simulink model "sm_robotic_wrist"  (R2021b)
settings: Solver=ode15s  StartTime=0.0  StopTime=10  FixedStep=1e-3  MaxStep=0.1  RelTol=1e-4  AbsTol=1e-4  EnableMultiTasking=on
model workspace: external: MATLAB File sm_robotic_wrist_params.m (data not in the file)
values from neighbouring files (symbols this model uses):
  Ca = 60    [sm_robotic_wrist_params.m]
  color = simmechanics.demohelpers.colors    [sm_robotic_wrist_params.m]
  density = simmechanics.demohelpers.densities    [sm_robotic_wrist_params.m]
undefined symbols (not defined in the file or in its folder): forearm, prcarrier, prshaft, tassm, trcarrier, trshaft, wshaft, X, Y, Z
libraries: sm_lib x44, sm_robotic_wrist_lib x12, nesl_utility x4
(part 1 of 2)
Description:
  | 3-Roll Robotic Wrist Mechanism
  | 
  | This example models a 3-Roll robotic wrist mechanism based on the Cincinnati-Milacron 3-roll wrist mechanism. The mechanism uses three bevel gear pairs to rotate the tool about 3 independent axes. The tip of the tool moves along the surface of a sphere and can be rotated about an axis that passes through the center of that sphere (drilling action). In this example, precomputed torques are applied to the three drive shafts to achieve a certain trajectory (on the surface of the sphere) of the tool tip. Drilling is performed at different points along the trajectory.
settings Model: Creator=The MathWorks, Inc.  LastModifiedBy=The MathWorks, Inc.
settings SolverCC: AutoScaleAbsTol=off  AlgebraicLoopSolver=TrustRegion
settings DataIOCC: LimitDataPoints=on  SaveFormat=Array  SaveOutput=off  SaveTime=off  ReturnWorkspaceOutputs=off
settings OptimizationCC: LifeSpan=inf
settings DebuggingCC: UnderspecifiedInitializationDetection=Classic  MergeDetectMultiDrivingBlocksExec=none  SFUnexpectedBacktrackingDiag=warning  SFNoUnconditionalDefaultTransitionDiag=warning  SFExecutionAtInitializationDiag=none  SFMachineParentedDataDiag=warning  ArithmeticOperatorsInVariantConditions=warning
settings HardwareCC: ProdBitPerPointer=32  ProdBitPerSizeT=32  ProdBitPerPtrDiffT=32  ProdLargestAtomicFloat=None  ProdIntDivRoundTo=Undefined  ProdEndianess=Unspecified  ProdWordSize=32  ProdHWDeviceType=32-bit Generic
settings ModelReferenceCC: PropagateSignalLabelsOutOfModel=off
settings SFSimCC: SimUseLocalCustomCode=off  CustomCodeUndefinedFunction=UseInterfaceOnly
settings RTWCC: RTWUseLocalCustomCode=off
settings CodeAppCC: StateflowObjectComments=on
settings GRTTargetCC: TargetLangStandard=C89/C90 (ANSI)
settings ConfigComp: CovMetricSettings=dw  CovSaveCumulativeToWorkspaceVar=on  CovSaveSingleToWorkspaceVar=on  CovExternalEMLEnable=off
settings SimscapeCC: SimscapeNormalizeSystem=off
settings ConfigurationSet: Description=SimMechanics 2G
settings ExplorerConfigSet: InternalSimMechanicsExplorerSettings="<ExplorerConfiguration><canonicalview>default</canonicalview><TilePanel><TileInfo><Tiles Columns=\"1\" Count=\"1\" Rows=\"1\"><Column Left=\"2\" Weight=\"1\"/><Column Left=\"812\"/><Row Top=\"2\" Weight=\"1\"/><Row Top=\"689\"/><Tile Height=\"1\" Width=\"1\" X=\"0\" Y=\"0\"/></Tiles></TileInfo><SceneInfo><SceneViewer><BGColor><R>0.60000002384185791</R><G>0.60000002384185791</G><B>0.60000002384185791</B></BGColor><Camera><Position><X>0.167588576674461365</X><Y>-0.43597028678660954</Y><Z>1.21854245662689209e-05</Z></Position><Center><X>0.167588576674461365</X><Y>1.28261744976043701e-05</Y><Z>1.21854245662689209e-05</Z></Center><Up><X>0</X><Y>-0</Y><Z>1</Z></Up><Left>-0.17596800550818445</Left><Right>0.17596800550818445</Right><Bottom>-0.0837415538728237124</Bottom><Top>0.0837415538728237124</Top></Camera></SceneViewer></SceneInfo></TilePanel></ExplorerConfiguration>"

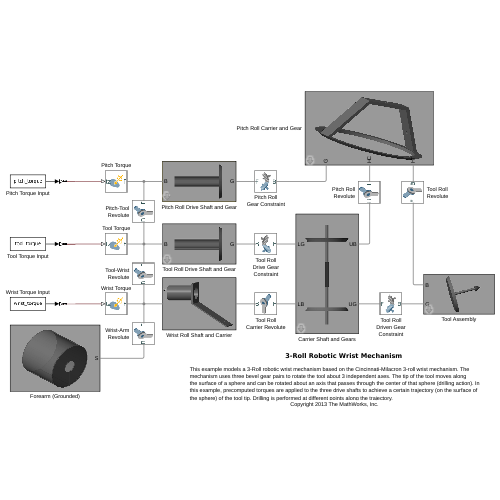
[thumbnail: Simulink's stored preview of the top-level diagram]
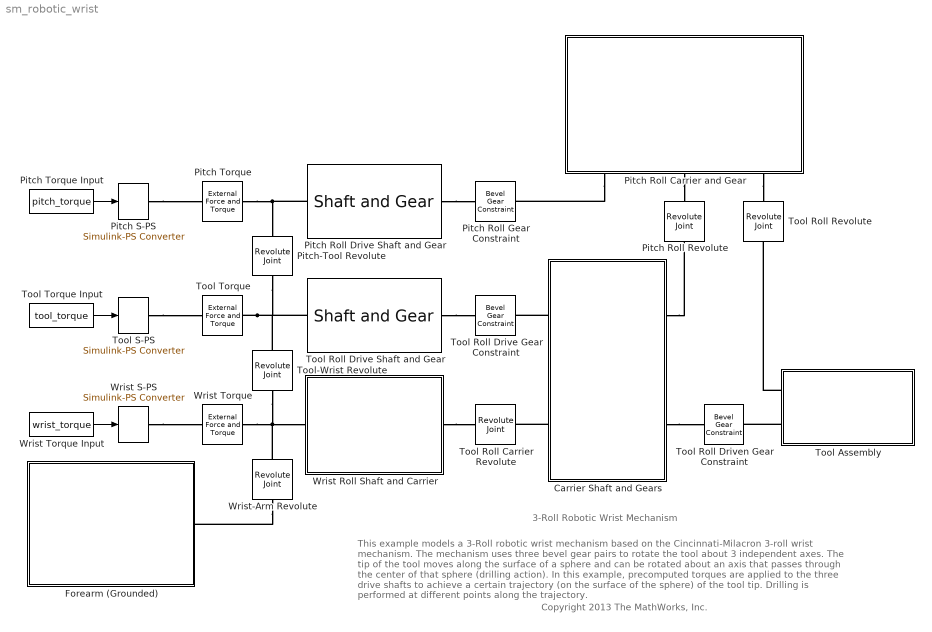
== system sm_robotic_wrist ==
  note: 3-Roll Robotic Wrist Mechanism
  note: Copyright 2013 The MathWorks, Inc.
  note: This example models a 3-Roll robotic wrist mechanism based on the Cincinnati-Milacron 3-roll wrist mechanism. The
      | mechanism uses three bevel gear pairs to rotate the tool about 3 independent axes. The tip of the tool moves along
      | the surface of a sphere and can be rotated about an axis that passes through the center of that sphere (drilling action). In
      | this example, precomputed torques are applied to the three drive shafts to achieve a certain trajectory (on the surface of
      | the sphere) of the tool tip. Drilling is performed at different points along the trajectory.
  Carrier Shaft and Gears : Subsystem  mask(Tool Roll Carrier){R=trcarrier.Rs, L=trcarrier.Ls, Og=trcarrier.Og, Ohl=trcarrier.Olb, Ohu=trcarrier.Oub, Rg=trcarrier.Rg, Tg=trcarrier.Tg, Ca=90-Ca, Hg=trcarrier.Rgh, rho=density.aluminum, clr=color.yellow}
      mask prompts: R "Radius (cm):"; L "Length (cm):"; Og "Gear offset (cm):"; Ohl "Lower hinge offset (cm):"; Ohu "Upper hinge offset (cm):"; Rg "Gear radius (cm):"; Tg "Gear thickness (cm):"; Ca "Gear cone angle (deg):"; Hg "Gear hole radius (cm):"; rho "Density (kg/m^3)"; clr "Color [r g b]:"
      mask help:
      | This block models the intermediate carrier (with bevel gears) that transmits the torque from the tool roll drive shaft to the tool.
      |
      | The port LG and UG correspond to the frames of the lower and upper gears.
      |
      | The port LB and UB correspond to the frames of the lower and upper bearing points.
      mask DialogControl Container4 Prompt: Shaft
      mask DialogControl Container4_copy_copy Prompt: Gears
      mask DialogControl Container4_copy Prompt: Material Properties
      mask Display:
      | image(fullfile(matlabroot,'toolbox','physmod','sm','smdemos','robotic_wrist','images','sm_rwrist_toolrollcarrier.png'))
      | port_label('LConn',1,'LG')
      | port_label('LConn',2,'LB')
      | port_label('RConn',1,'UB')
      | port_label('RConn',2,'UG')
  Forearm (Grounded) : Subsystem
      mask Display:
      | image(fullfile(matlabroot,'toolbox','physmod','sm','smdemos','robotic_wrist','images','sm_rwrist_forearm.png'))
      | port_label('RConn',1,'S')
  Pitch Roll Gear Constraint : sm_lib/Gears and Couplings/Gears/Bevel Gear Constraint  BaseGearRadius=prcarrier.Rg  BaseGearRadiusUnits=cm  FollGearRadius=prshaft.Rg  FollGearRadiusUnits=cm  AssemblyGearRotation=Free  ShaftOrientation=ArbitrarilyOriented  ShaftAngle=180-Ca  ShaftAngleUnits=deg
      settings: SourceProductBaseCode=MS
  Pitch Roll Revolute : sm_lib/Joints/Revolute Joint  JointMode=Normal  SenseConstraintForce=off  SenseConstraintForceX=off  SenseConstraintForceY=off  SenseConstraintForceZ=off  SenseConstraintTorque=off  SenseConstraintTorqueX=off  SenseConstraintTorqueY=off  SenseConstraintTorqueZ=off  SenseTotalForce=off  SenseTotalForceX=off  SenseTotalForceY=off  SenseTotalForceZ=off  SenseTotalTorque=off  SenseTotalTorqueX=off  SenseTotalTorqueY=off  SenseTotalTorqueZ=off  CompositeWrenchDir=FollowerOnBase  CompositeWrenchFrame=BaseFrame  EquilibriumPosition=0  EquilibriumPositionUnits=deg  SpringStiffness=0  SpringStiffnessUnits=N*m/deg  DampingCoefficient=0  DampingCoefficientUnits=N*m/(deg/s)  TorqueActuationMode=NoTorque  MotionActuationMode=ComputedMotion  SensePosition=off  SenseVelocity=off  SenseAcceleration=off  SenseTorqueForce=off  SenseLowerLimitTorqueForce=off  SenseUpperLimitTorqueForce=off  LowerLimitSpecify=off  LowerLimitBound=-90  LowerLimitBoundUnits=deg  LowerLimitStiffness=1e4  LowerLimitStiffnessUnits=N*m/deg  LowerLimitDamping=10  LowerLimitDampingUnits=N*m/(deg/s)  LowerLimitTransitionRegionWidth=0.1  LowerLimitTransitionRegionWidthUnits=deg  UpperLimitSpecify=off  UpperLimitBound=90  UpperLimitBoundUnits=deg  UpperLimitStiffness=1e4  UpperLimitStiffnessUnits=N*m/deg  UpperLimitDamping=10  UpperLimitDampingUnits=N*m/(deg/s)  UpperLimitTransitionRegionWidth=0.1  UpperLimitTransitionRegionWidthUnits=deg  PositionTargetSpecify=on  PositionTargetPriority=High  PositionTargetValue=joint_targets.pitch_roll.q  PositionTargetValueUnits=rad  VelocityTargetSpecify=on  VelocityTargetPriority=High  VelocityTargetValue=joint_targets.pitch_roll.w  VelocityTargetValueUnits=rad/s
  Pitch Roll Carrier and Gear : Subsystem  mask(Pitch Roll Carrier){Hc=prcarrier.Hc, Ac=Ca, Tc=prcarrier.Tc, Wc=prcarrier.Wc, Rht=prcarrier.Rht, Rhc=prcarrier.Rhc, Rg=prcarrier.Rg, Tg=prcarrier.Tg, Rgh=prcarrier.Rgh, Ag=Ca, rho=density.aluminum, cclr=color.brown, gclr=color.brown}
      mask prompts: Hc "Carrier height (cm):"; Ac "Carrier arms angle (deg):"; Tc "Carrier arms thickness (cm):"; Wc "Carrier arms width (cm):"; Rht "Tool shaft hole radius (cm):"; Rhc "Carrier shaft hole radius (cm):"; Rg "Gear radius (cm):"; Tg "Gear thickness (cm):"; Rgh "Gear hole radius (cm):"; Ag "Gear cone angle (deg):"; rho "Density (kg/m^3):"; cclr "Carrier color [r g b]:"; gclr "Gear color [r g b]:"
      mask help:
      | This block models the pitch roll carrier and gear that carries the tool and rotates the tool about the pitch axis. The bevel gear is welded to the carrier and is driven by the pitch roll drive shaft.
      |
      | The port G corresponds to the center of the bevel gear.
      |
      | The port HC corresponds to the bearing between the pitch carrier and the tool roll carrier.
      |
      | The port HT correponds to the bearing between the pitch carrier and the tool assembly.
      mask init:
      | sn = sin(Ac*pi/180);
      | tn = tan(Ac*pi/180);
      | 
      | sn1 = sin((90-Ac)*pi/180);
      | cn1 = cos((90-Ac)*pi/180);
      | 
      | w = Tc/sn;
      | Oht = (Hc-Tc)/sn - (Rg-w/2)*sn1 + Tg*sn/2;
      | 
      | carrier_left_xsec = [-2*Rhc             Hc
      |                     -Rg-w/2+Hc/tn      Hc;
      |                     -Rg-w/2            0;
      |                     -Rg+w/2            0;
      |                     -Rg+w/2+(Hc-Tc)/tn Hc-Tc;
      |                     -2*Rhc             Hc-Tc];
      |                 
      | carrier_right_top_xsec = ...
      |      [2*Rhc                                     Hc-Tc;
      |       Rg-w/2-(Hc-Tc)/tn                         Hc-Tc;
      |       Rg-w/2-(Hc-Tc)/tn+(Oht-2*Rht)*sn1         Hc-Tc-(Oht-2*Rht)*cn1;
      |       Rg-w/2-(Hc-Tc)/tn+(Oht-2*Rht)*sn1+Tc*cn1  Hc-Tc-(Oht-2*Rht)*cn1+Tc*sn1;
      |       Rg+w/2-Hc/tn                              Hc;
      |       2*Rhc                                     Hc
      |      ];
      |    
      | carrier_right_bot_xsec = ...
      |       [ Rg-w/2                                    0;
      |         Rg+w/2                                    0;
      |         Rg-w/2-(Hc-Tc)/tn+(Oht+2*Rht)*sn1+Tc*cn1  Hc-Tc-(Oht+2*Rht)*cn1+Tc*sn1;
      |         Rg-w/2-(Hc-Tc)/tn+(Oht+2*Rht)*sn1         Hc-Tc-(Oht+2*Rht)*cn1
      |       ];
      |   
      | rhx = Rg-w/2-(Hc-Tc)/tn+Oht*sn1;
      | rhy = Hc-Tc -Oht*cn1;
      mask DialogControl Container4 Prompt: Carrier Arm
      mask DialogControl Container4_copy Prompt: Gear
      mask DialogControl Container4_copy_copy Prompt: Material Properties
      mask Display:
      | image(fullfile(matlabroot,'toolbox','physmod','sm','smdemos','robotic_wrist','images','sm_rwrist_pitchrollcarrier.png'))
      | port_label('RConn',1,'G')
      | port_label('RConn',2,'HC')
      | port_label('RConn',3,'HT')
  Pitch Roll Drive Shaft and Gear : sm_robotic_wrist_lib/Shaft and Gear  L=prshaft.Ls  Ro=prshaft.Rso  Ri=prshaft.Rsi  Rg=prshaft.Rg  Tg=prshaft.Tg  Cag=Ca  rho=density.aluminum  clr=color.brown  Os=1
      settings: SourceProductBaseCode=MS
  Pitch S-PS : nesl_utility/Simulink-PS Converter  PhysicalDomain=network_engine_domain  SubClassName=ps_input  LeftPortType=input  RightPortType=output  PseudoPeriodic=off  Frequencies=[]  NoiseDistribution=none  NoiseParameters=[]  Unit=1  AffineConversion=off  FilteringAndDerivatives=filter  SimscapeFilterOrder=2  InputFilterTimeConstant=0.01  UdotUserProvided=1
      settings: SourceProductBaseCode=PW,SS
  Pitch Torque : sm_lib/Forces and Torques/External Force and Torque  ForceResolutionFrame=AttachedFrame  EnableForceX=off  EnableForceY=off  EnableForceZ=off  EnableForce=off  TorqueResolutionFrame=AttachedFrame  EnableTorqueX=off  EnableTorqueY=off  EnableTorqueZ=on  EnableTorque=off
  Pitch Torque Input : FromWorkspace  VariableName=pitch_torque
  Pitch-Tool Revolute : sm_lib/Joints/Revolute Joint  JointMode=Normal  SenseConstraintForce=off  SenseConstraintForceX=off  SenseConstraintForceY=off  SenseConstraintForceZ=off  SenseConstraintTorque=off  SenseConstraintTorqueX=off  SenseConstraintTorqueY=off  SenseConstraintTorqueZ=off  SenseTotalForce=off  SenseTotalForceX=off  SenseTotalForceY=off  SenseTotalForceZ=off  SenseTotalTorque=off  SenseTotalTorqueX=off  SenseTotalTorqueY=off  SenseTotalTorqueZ=off  CompositeWrenchDir=FollowerOnBase  CompositeWrenchFrame=BaseFrame  EquilibriumPosition=0  EquilibriumPositionUnits=deg  SpringStiffness=0  SpringStiffnessUnits=N*m/deg  DampingCoefficient=5e-3  DampingCoefficientUnits=N*m/(deg/s)  TorqueActuationMode=NoTorque  MotionActuationMode=ComputedMotion  SensePosition=off  SenseVelocity=off  SenseAcceleration=off  SenseTorqueForce=off  SenseLowerLimitTorqueForce=off  SenseUpperLimitTorqueForce=off  LowerLimitSpecify=off  LowerLimitBound=-90  LowerLimitBoundUnits=deg  LowerLimitStiffness=1e4  LowerLimitStiffnessUnits=N*m/deg  LowerLimitDamping=10  LowerLimitDampingUnits=N*m/(deg/s)  LowerLimitTransitionRegionWidth=0.1  LowerLimitTransitionRegionWidthUnits=deg  UpperLimitSpecify=off  UpperLimitBound=90  UpperLimitBoundUnits=deg  UpperLimitStiffness=1e4  UpperLimitStiffnessUnits=N*m/deg  UpperLimitDamping=10  UpperLimitDampingUnits=N*m/(deg/s)  UpperLimitTransitionRegionWidth=0.1  UpperLimitTransitionRegionWidthUnits=deg  PositionTargetSpecify=on  PositionTargetPriority=High  PositionTargetValue=joint_targets.pitch_tool.q  PositionTargetValueUnits=rad  VelocityTargetSpecify=on  VelocityTargetPriority=High  VelocityTargetValue=joint_targets.pitch_tool.w  VelocityTargetValueUnits=rad/s
  Tool Assembly : Subsystem  mask(Tool Assembly){L=tassm.Ls, R=tassm.Rs, Oh=tassm.Ohs, Rd=tassm.Rd, Hd=tassm.Hd, Rg=tassm.Rg, Tg=tassm.Tg, Cag=90-Ca, rho=density.aluminum, clr=color.yellow}
      mask prompts: L "Shaft length (cm):"; R "Shaft radius (cm):"; Oh "Hinge offset (cm):"; Rd "Drill base radius (cm):"; Hd "Drill height (cm):"; Rg "Gear radius (cm):"; Tg "Gear thickness (cm):"; Cag "Gear cone angle (deg):"; rho "Density (kg/m^3):"; clr "Color [r g b]:"
      mask help:
      | This block models the drill tool and the attached bevel gear. The bevel gear is driven by the tool roll gear train.
      |
      | The port G corresponds to the frame at the center of the bevel gear.
      |
      | The port B corresponds to the frame at the pitch roll carrier bearing.
      mask init:
      | drill_xsec = [0 0; Rd 0; 0 Hd];
      mask DialogControl Container4 Prompt: Tool
      mask DialogControl Container4_copy Prompt: Gear
      mask DialogControl Container4_copy_copy Prompt: Material Properties
      mask Display:
      | image(fullfile(matlabroot,'toolbox','physmod','sm','smdemos','robotic_wrist','images','sm_rwrist_toolassm.png'))
      | port_label('LConn',1,'B')
      | port_label('LConn',2,'G')
  Tool Roll Carrier Revolute : sm_lib/Joints/Revolute Joint  JointMode=Normal  SenseConstraintForce=off  SenseConstraintForceX=off  SenseConstraintForceY=off  SenseConstraintForceZ=off  SenseConstraintTorque=off  SenseConstraintTorqueX=off  SenseConstraintTorqueY=off  SenseConstraintTorqueZ=off  SenseTotalForce=off  SenseTotalForceX=off  SenseTotalForceY=off  SenseTotalForceZ=off  SenseTotalTorque=off  SenseTotalTorqueX=off  SenseTotalTorqueY=off  SenseTotalTorqueZ=off  CompositeWrenchDir=FollowerOnBase  CompositeWrenchFrame=BaseFrame  EquilibriumPosition=0  EquilibriumPositionUnits=deg  SpringStiffness=0  SpringStiffnessUnits=N*m/deg  DampingCoefficient=0  DampingCoefficientUnits=N*m/(deg/s)  TorqueActuationMode=NoTorque  MotionActuationMode=ComputedMotion  SensePosition=off  SenseVelocity=off  SenseAcceleration=off  SenseTorqueForce=off  SenseLowerLimitTorqueForce=off  SenseUpperLimitTorqueForce=off  LowerLimitSpecify=off  LowerLimitBound=-90  LowerLimitBoundUnits=deg  LowerLimitStiffness=1e4  LowerLimitStiffnessUnits=N*m/deg  LowerLimitDamping=10  LowerLimitDampingUnits=N*m/(deg/s)  LowerLimitTransitionRegionWidth=0.1  LowerLimitTransitionRegionWidthUnits=deg  UpperLimitSpecify=off  UpperLimitBound=90  UpperLimitBoundUnits=deg  UpperLimitStiffness=1e4  UpperLimitStiffnessUnits=N*m/deg  UpperLimitDamping=10  UpperLimitDampingUnits=N*m/(deg/s)  UpperLimitTransitionRegionWidth=0.1  UpperLimitTransitionRegionWidthUnits=deg  PositionTargetSpecify=off  PositionTargetPriority=High  PositionTargetValue=-2.786559909696359e+00  PositionTargetValueUnits=deg  VelocityTargetSpecify=off  VelocityTargetPriority=High  VelocityTargetValue=0  VelocityTargetValueUnits=deg/s
  Tool Roll Drive Gear Constraint : sm_lib/Gears and Couplings/Gears/Bevel Gear Constraint  BaseGearRadius=trshaft.Rg  BaseGearRadiusUnits=cm  FollGearRadius=trcarrier.Rg  FollGearRadiusUnits=cm  AssemblyGearRotation=Free  ShaftOrientation=ArbitrarilyOriented  ShaftAngle=Ca  ShaftAngleUnits=deg
      settings: SourceProductBaseCode=MS
  Tool Roll Driven Gear Constraint : sm_lib/Gears and Couplings/Gears/Bevel Gear Constraint  BaseGearRadius=tassm.Rg  BaseGearRadiusUnits=cm  FollGearRadius=trcarrier.Rg  FollGearRadiusUnits=cm  AssemblyGearRotation=Free  ShaftOrientation=ArbitrarilyOriented  ShaftAngle=Ca  ShaftAngleUnits=deg
      settings: SourceProductBaseCode=MS
  Tool Roll Revolute : sm_lib/Joints/Revolute Joint  JointMode=Normal  SenseConstraintForce=off  SenseConstraintForceX=off  SenseConstraintForceY=off  SenseConstraintForceZ=off  SenseConstraintTorque=off  SenseConstraintTorqueX=off  SenseConstraintTorqueY=off  SenseConstraintTorqueZ=off  SenseTotalForce=off  SenseTotalForceX=off  SenseTotalForceY=off  SenseTotalForceZ=off  SenseTotalTorque=off  SenseTotalTorqueX=off  SenseTotalTorqueY=off  SenseTotalTorqueZ=off  CompositeWrenchDir=FollowerOnBase  CompositeWrenchFrame=BaseFrame  EquilibriumPosition=0  EquilibriumPositionUnits=deg  SpringStiffness=0  SpringStiffnessUnits=N*m/deg  DampingCoefficient=0  DampingCoefficientUnits=N*m/(deg/s)  TorqueActuationMode=NoTorque  MotionActuationMode=ComputedMotion  SensePosition=off  SenseVelocity=off  SenseAcceleration=off  SenseTorqueForce=off  SenseLowerLimitTorqueForce=off  SenseUpperLimitTorqueForce=off  LowerLimitSpecify=off  LowerLimitBound=-90  LowerLimitBoundUnits=deg  LowerLimitStiffness=1e4  LowerLimitStiffnessUnits=N*m/deg  LowerLimitDamping=10  LowerLimitDampingUnits=N*m/(deg/s)  LowerLimitTransitionRegionWidth=0.1  LowerLimitTransitionRegionWidthUnits=deg  UpperLimitSpecify=off  UpperLimitBound=90  UpperLimitBoundUnits=deg  UpperLimitStiffness=1e4  UpperLimitStiffnessUnits=N*m/deg  UpperLimitDamping=10  UpperLimitDampingUnits=N*m/(deg/s)  UpperLimitTransitionRegionWidth=0.1  UpperLimitTransitionRegionWidthUnits=deg  PositionTargetSpecify=off  PositionTargetPriority=High  PositionTargetValue=-4.321120546852593e+01  PositionTargetValueUnits=deg  VelocityTargetSpecify=off  VelocityTargetPriority=High  VelocityTargetValue=0  VelocityTargetValueUnits=deg/s
  Tool Roll Drive Shaft and Gear : sm_robotic_wrist_lib/Shaft and Gear  L=trshaft.Ls  Ro=trshaft.Rso  Ri=trshaft.Rsi  Rg=trshaft.Rg  Tg=trshaft.Tg  Cag=90-Ca  rho=density.aluminum  clr=color.yellow  Os=1
      settings: SourceProductBaseCode=MS
  Tool S-PS : nesl_utility/Simulink-PS Converter  PhysicalDomain=network_engine_domain  SubClassName=ps_input  LeftPortType=input  RightPortType=output  PseudoPeriodic=off  Frequencies=[]  NoiseDistribution=none  NoiseParameters=[]  Unit=1  AffineConversion=off  FilteringAndDerivatives=filter  SimscapeFilterOrder=2  InputFilterTimeConstant=0.01  UdotUserProvided=1
      settings: SourceProductBaseCode=PW,SS
  Tool Torque : sm_lib/Forces and Torques/External Force and Torque  ForceResolutionFrame=AttachedFrame  EnableForceX=off  EnableForceY=off  EnableForceZ=off  EnableForce=off  TorqueResolutionFrame=AttachedFrame  EnableTorqueX=off  EnableTorqueY=off  EnableTorqueZ=on  EnableTorque=off
  Tool Torque Input : FromWorkspace  VariableName=tool_torque
  Tool-Wrist Revolute : sm_lib/Joints/Revolute Joint  JointMode=Normal  SenseConstraintForce=off  SenseConstraintForceX=off  SenseConstraintForceY=off  SenseConstraintForceZ=off  SenseConstraintTorque=off  SenseConstraintTorqueX=off  SenseConstraintTorqueY=off  SenseConstraintTorqueZ=off  SenseTotalForce=off  SenseTotalForceX=off  SenseTotalForceY=off  SenseTotalForceZ=off  SenseTotalTorque=off  SenseTotalTorqueX=off  SenseTotalTorqueY=off  SenseTotalTorqueZ=off  CompositeWrenchDir=FollowerOnBase  CompositeWrenchFrame=BaseFrame  EquilibriumPosition=0  EquilibriumPositionUnits=deg  SpringStiffness=0  SpringStiffnessUnits=N*m/deg  DampingCoefficient=5e-3  DampingCoefficientUnits=N*m/(deg/s)  TorqueActuationMode=NoTorque  MotionActuationMode=ComputedMotion  SensePosition=off  SenseVelocity=off  SenseAcceleration=off  SenseTorqueForce=off  SenseLowerLimitTorqueForce=off  SenseUpperLimitTorqueForce=off  LowerLimitSpecify=off  LowerLimitBound=-90  LowerLimitBoundUnits=deg  LowerLimitStiffness=1e4  LowerLimitStiffnessUnits=N*m/deg  LowerLimitDamping=10  LowerLimitDampingUnits=N*m/(deg/s)  LowerLimitTransitionRegionWidth=0.1  LowerLimitTransitionRegionWidthUnits=deg  UpperLimitSpecify=off  UpperLimitBound=90  UpperLimitBoundUnits=deg  UpperLimitStiffness=1e4  UpperLimitStiffnessUnits=N*m/deg  UpperLimitDamping=10  UpperLimitDampingUnits=N*m/(deg/s)  UpperLimitTransitionRegionWidth=0.1  UpperLimitTransitionRegionWidthUnits=deg  PositionTargetSpecify=on  PositionTargetPriority=High  PositionTargetValue=joint_targets.tool_wrist.q  PositionTargetValueUnits=rad  VelocityTargetSpecify=on  VelocityTargetPriority=High  VelocityTargetValue=joint_targets.tool_wrist.w  VelocityTargetValueUnits=rad/s
  Wrist Roll Shaft and Carrier : Subsystem
      mask Display: image(fullfile(matlabroot,'toolbox','physmod','sm','smdemos','robotic_wrist','images','sm_rwrist_wristshaftcarrier.png'))
  Wrist S-PS : nesl_utility/Simulink-PS Converter  PhysicalDomain=network_engine_domain  SubClassName=ps_input  LeftPortType=input  RightPortType=output  PseudoPeriodic=off  Frequencies=[]  NoiseDistribution=none  NoiseParameters=[]  Unit=1  AffineConversion=off  FilteringAndDerivatives=filter  SimscapeFilterOrder=2  InputFilterTimeConstant=0.01  UdotUserProvided=1
      settings: SourceProductBaseCode=PW,SS
  Wrist Torque : sm_lib/Forces and Torques/External Force and Torque  ForceResolutionFrame=AttachedFrame  EnableForceX=off  EnableForceY=off  EnableForceZ=off  EnableForce=off  TorqueResolutionFrame=AttachedFrame  EnableTorqueX=off  EnableTorqueY=off  EnableTorqueZ=on  EnableTorque=off
  Wrist Torque Input : FromWorkspace  VariableName=wrist_torque
  Wrist-Arm Revolute : sm_lib/Joints/Revolute Joint  JointMode=Normal  SenseConstraintForce=off  SenseConstraintForceX=off  SenseConstraintForceY=off  SenseConstraintForceZ=off  SenseConstraintTorque=off  SenseConstraintTorqueX=off  SenseConstraintTorqueY=off  SenseConstraintTorqueZ=off  SenseTotalForce=off  SenseTotalForceX=off  SenseTotalForceY=off  SenseTotalForceZ=off  SenseTotalTorque=off  SenseTotalTorqueX=off  SenseTotalTorqueY=off  SenseTotalTorqueZ=off  CompositeWrenchDir=FollowerOnBase  CompositeWrenchFrame=BaseFrame  EquilibriumPosition=0  EquilibriumPositionUnits=deg  SpringStiffness=0  SpringStiffnessUnits=N*m/deg  DampingCoefficient=5e-3  DampingCoefficientUnits=N*m/(deg/s)  TorqueActuationMode=NoTorque  MotionActuationMode=ComputedMotion  SensePosition=off  SenseVelocity=off  SenseAcceleration=off  SenseTorqueForce=off  SenseLowerLimitTorqueForce=off  SenseUpperLimitTorqueForce=off  LowerLimitSpecify=off  LowerLimitBound=-90  LowerLimitBoundUnits=deg  LowerLimitStiffness=1e4  LowerLimitStiffnessUnits=N*m/deg  LowerLimitDamping=10  LowerLimitDampingUnits=N*m/(deg/s)  LowerLimitTransitionRegionWidth=0.1  LowerLimitTransitionRegionWidthUnits=deg  UpperLimitSpecify=off  UpperLimitBound=90  UpperLimitBoundUnits=deg  UpperLimitStiffness=1e4  UpperLimitStiffnessUnits=N*m/deg  UpperLimitDamping=10  UpperLimitDampingUnits=N*m/(deg/s)  UpperLimitTransitionRegionWidth=0.1  UpperLimitTransitionRegionWidthUnits=deg  PositionTargetSpecify=on  PositionTargetPriority=High  PositionTargetValue=joint_targets.wrist_arm.q  PositionTargetValueUnits=rad  VelocityTargetSpecify=on  VelocityTargetPriority=High  VelocityTargetValue=joint_targets.wrist_arm.w  VelocityTargetValueUnits=rad/s
  wires:
  Pitch Torque Input/1 -> Pitch S-PS/1
  Wrist Torque Input/1 -> Wrist S-PS/1
  Tool Torque Input/1 -> Tool S-PS/1
  connections:
  Wrist Torque/RConn1 -- Wrist-Arm Revolute/RConn1 -- Wrist Roll Shaft and Carrier/LConn1 -- Tool-Wrist Revolute/LConn1
  Pitch Torque/RConn1 -- Pitch Roll Drive Shaft and Gear/LConn1 -- Pitch-Tool Revolute/RConn1
  Tool Torque/RConn1 -- Tool Roll Drive Shaft and Gear/LConn1 -- Pitch-Tool Revolute/LConn1 -- Tool-Wrist Revolute/RConn1
  Carrier Shaft and Gears/LConn2 -- Tool Roll Carrier Revolute/RConn1
  Pitch Roll Carrier and Gear/RConn2 -- Pitch Roll Revolute/RConn1
  Pitch Roll Carrier and Gear/RConn1 -- Pitch Roll Gear Constraint/LConn1
  Pitch Roll Carrier and Gear/RConn3 -- Tool Roll Revolute/LConn1
  Wrist-Arm Revolute/LConn1 -- Forearm (Grounded)/RConn1
  Tool Roll Drive Shaft and Gear/RConn1 -- Tool Roll Drive Gear Constraint/LConn1
  Carrier Shaft and Gears/RConn2 -- Tool Roll Driven Gear Constraint/RConn1
  Carrier Shaft and Gears/RConn1 -- Pitch Roll Revolute/LConn1
  Wrist Roll Shaft and Carrier/RConn1 -- Tool Roll Carrier Revolute/LConn1
  Pitch S-PS/RConn1 -- Pitch Torque/LConn1
  Wrist S-PS/RConn1 -- Wrist Torque/LConn1
  Carrier Shaft and Gears/LConn1 -- Tool Roll Drive Gear Constraint/RConn1
  Tool S-PS/RConn1 -- Tool Torque/LConn1
  Tool Assembly/LConn2 -- Tool Roll Driven Gear Constraint/LConn1
  Tool Assembly/LConn1 -- Tool Roll Revolute/RConn1
  Pitch Roll Drive Shaft and Gear/RConn1 -- Pitch Roll Gear Constraint/RConn1

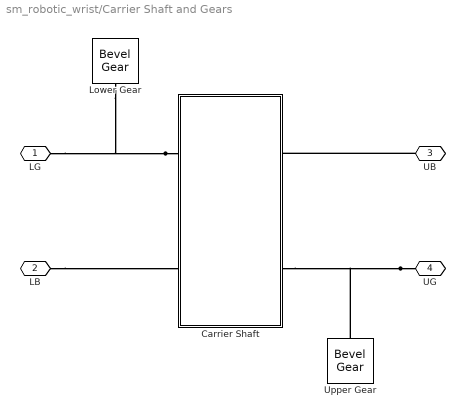
== system sm_robotic_wrist/Carrier Shaft and Gears ==
  Carrier Shaft : Subsystem
      mask Display:
      | image(fullfile(matlabroot,'toolbox','physmod','sm','smdemos','robotic_wrist','images','sm_rwrist_tcarriershaft.png'))
      | port_label('LConn',1,'LG')
      | port_label('LConn',2,'LB')
      | port_label('RConn',1,'UB')
      | port_label('RConn',2,'UG')
  Lower Gear : sm_robotic_wrist_lib/Bevel Gear  R=Rg  T=Tg  Ca=Ca  Rh=Hg  rho=rho  clr=clr
      settings: SourceProductBaseCode=MS
  Upper Gear : sm_robotic_wrist_lib/Bevel Gear  R=Rg  T=Tg  Ca=Ca  Rh=Hg  rho=rho  clr=clr
      settings: SourceProductBaseCode=MS
  LG : PMIOPort  Side=Left
  LB : PMIOPort  Port=2  Side=Left
  UB : PMIOPort  Port=3  Side=Right
  UG : PMIOPort  Port=4  Side=Right
  connections:
  Carrier Shaft/LConn1 -- Lower Gear/LConn1 -- LG/RConn1
  UG/RConn1 -- Upper Gear/LConn1 -- Carrier Shaft/RConn2
  UB/RConn1 -- Carrier Shaft/RConn1
  LB/RConn1 -- Carrier Shaft/LConn2

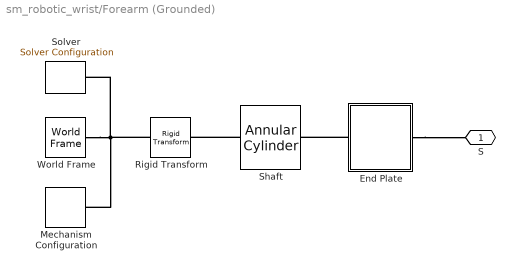
== system sm_robotic_wrist/Forearm (Grounded) ==
  End Plate : Subsystem  mask(Annular Cylinder){Ro=forearm.Ro, Ri=forearm.Rsh, L=forearm.Tep, rho=density.aluminum, clr=color.brown, opc=0.6}
      mask prompts: Ro "Cylinder outer radius (cm)"; Ri "Cylinder inner radius (cm)"; L "Cylinder length (cm)"; rho "Density (kg/m^3)"; clr "Color"; opc "Opacity"
      mask init:
      | theta = linspace(0,360,360)'*pi/180;
      | annular_sec = [Ro*cos(theta) Ro*sin(theta);
      |                Ri*cos(theta(end:-1:1)) Ri*sin(theta(end:-1:1))];
      mask Display: image('sm_wlandgear_acyl.png');
  Mechanism Configuration : sm_lib/Utilities/Mechanism Configuration  UniformGravity=Constant  GravityVector=[0 0 -9.81]  GravityUnits=m/s^2  LinearizationDelta=0.001  JointModeTransitionNonlinearIterations=2
  Rigid Transform : sm_lib/Frames and Transforms/Rigid Transform  TranslationMethod=None  TranslationStandardOffset=0  TranslationLengthUnit=m  TranslationStandardAxis=+Z  TranslationCartesianOffset=[0 0 0]  TranslationROffset=0  TranslationROffsetUnits=m  TranslationZOffset=0  TranslationZOffsetUnits=m  TranslationThetaOffset=0  TranslationThetaOffsetUnits=deg  RotationMethod=AlignedAxes  RotationAngleUnits=deg  RotationStandardAxis=+Z  RotationAngle=0  RotationArbitraryAxis=[0 0 1]  FollAlignAxisA=+Z  BaseAlignAxisA=+X  FollAlignAxisB=+Y  BaseAlignAxisB=+Y  RotationSequenceAxes=FollowerAxes  RotationSequence=XYX  RotationSequenceAngles=[0 0 0]  RotationSequenceAnglesUnits=deg  RotationMatrix=[1 0 0; 0 1 0; 0 0 1]
  Shaft : sm_robotic_wrist_lib/Annular Cylinder  Ro=forearm.Ro  Ri=forearm.Ri  L=forearm.L  rho=density.aluminum  clr=color.brown  opc=0.6
      settings: SourceProductBaseCode=MS
  Solver : nesl_utility/Solver Configuration  PhysicalDomain=network_engine_domain  SubClassName=solver  LeftPortType=input  RightPortType=generic  Tones=[]  Harmonics=[]  SimulateNoise=off  Profile=off  UseLocalSampling=off  EnableSwitchedLinearOptims=on  FrequencyDomain=off  UseCCode=off  RelTol=0.001  AbsTol=1e-06  MinStep=1e-09  ToWorkspace=off  RevertToSquareIcSolve=off  NumHomotopyIterations=100  PhasorMode=off  PhasorModeNumHarmonics=1  DoDC=off  ResidualTolerance=1e-06  UseLocalSolver=off  LocalSolverChoice=NE_BACKWARD_EULER_ADVANCER  LocalSolverSampleTime=0.001  DoFixedCost=off  MaxNonlinIter=3  MaxModeIter=2  ComputeImpulses=off  ImpulseIterations=2  LinearAlgebra=Sparse  EquationFormulation=NE_TIME_EF  DelaysMemoryBudget=1024  AutomaticFiltering=on  FilteringTimeConstant=0.001  PartitionStorageMethod=AS_NEEDED  PartitionMemoryBudget=1024  PartitionMethod=FAST
      settings: SourceProductBaseCode=PW,SS
  World Frame : sm_lib/Frames and Transforms/World Frame
  S : PMIOPort  Side=Right
  connections:
  World Frame/RConn1 -- Rigid Transform/LConn1 -- Solver/RConn1 -- Mechanism Configuration/RConn1
  Shaft/LConn1 -- Rigid Transform/RConn1
  End Plate/LConn1 -- Shaft/RConn1
  End Plate/RConn1 -- S/RConn1

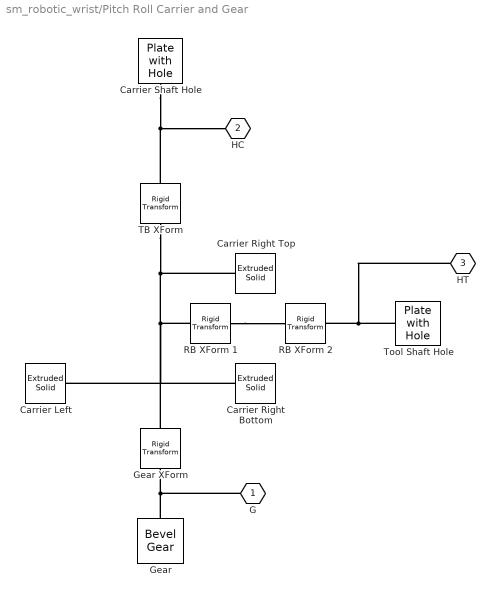
== system sm_robotic_wrist/Pitch Roll Carrier and Gear ==
  Carrier Left : sm_lib/Body Elements/Extruded Solid  GraphicAmbientColor=[0.15 0.15 0.15 1.0]  BasedOnType=Density  CenterOfMass=[0 0 0]  CenterOfMassUnits=m  GraphicDiffuseColor=cclr  ExportConvexHullGeometry=off  ExtrusionCrossSection=carrier_left_xsec  ExtrusionCrossSectionUnits=cm  Density=rho  DensityUnits=kg/(m^3)  DoExposeReferenceFrame=on  GraphicEmissiveColor=[0.0 0.0 0.0 1.0]  ExportEntireGeometry=off  ExtrusionLength=Wc  ExtrusionLengthUnits=cm  ExtrusionType=General  SerializedFrames=<Frames/>  MarkerShape=Sphere  MarkerSize=10  GraphicType=FromGeometry  InertiaType=CalculateFromGeometry  Mass=1  MassUnits=kg  MomentsOfInertia=[1 1 1]  MomentsOfInertiaUnits=kg*m^2  PolygonNumSides=3  GraphicOpacity=1.0  PolygonOuterRadius=1  PolygonOuterRadiusUnits=m  ProductsOfInertia=[0 0 0]  ProductsOfInertiaUnits=kg*m^2  GraphicShininess=75  GraphicSpecularColor=[0.5 0.5 0.5 1.0]  GraphicVisPropType=SimpleVisualProperties
  Carrier Right Bottom : sm_lib/Body Elements/Extruded Solid  GraphicAmbientColor=[0.15 0.15 0.15 1.0]  BasedOnType=Density  CenterOfMass=[0 0 0]  CenterOfMassUnits=m  GraphicDiffuseColor=cclr  ExportConvexHullGeometry=off  ExtrusionCrossSection=carrier_right_bot_xsec  ExtrusionCrossSectionUnits=cm  Density=rho  DensityUnits=kg/(m^3)  DoExposeReferenceFrame=on  GraphicEmissiveColor=[0.0 0.0 0.0 1.0]  ExportEntireGeometry=off  ExtrusionLength=Wc  ExtrusionLengthUnits=cm  ExtrusionType=General  SerializedFrames=<Frames/>  MarkerShape=Sphere  MarkerSize=10  GraphicType=FromGeometry  InertiaType=CalculateFromGeometry  Mass=1  MassUnits=kg  MomentsOfInertia=[1 1 1]  MomentsOfInertiaUnits=kg*m^2  PolygonNumSides=3  GraphicOpacity=1.0  PolygonOuterRadius=1  PolygonOuterRadiusUnits=m  ProductsOfInertia=[0 0 0]  ProductsOfInertiaUnits=kg*m^2  GraphicShininess=75  GraphicSpecularColor=[0.5 0.5 0.5 1.0]  GraphicVisPropType=SimpleVisualProperties
  Carrier Right Top : sm_lib/Body Elements/Extruded Solid  GraphicAmbientColor=[0.15 0.15 0.15 1.0]  BasedOnType=Density  CenterOfMass=[0 0 0]  CenterOfMassUnits=m  GraphicDiffuseColor=cclr  ExportConvexHullGeometry=off  ExtrusionCrossSection=carrier_right_top_xsec  ExtrusionCrossSectionUnits=cm  Density=rho  DensityUnits=kg/(m^3)  DoExposeReferenceFrame=on  GraphicEmissiveColor=[0.0 0.0 0.0 1.0]  ExportEntireGeometry=off  ExtrusionLength=Wc  ExtrusionLengthUnits=cm  ExtrusionType=General  SerializedFrames=<Frames/>  MarkerShape=Sphere  MarkerSize=10  GraphicType=FromGeometry  InertiaType=CalculateFromGeometry  Mass=1  MassUnits=kg  MomentsOfInertia=[1 1 1]  MomentsOfInertiaUnits=kg*m^2  PolygonNumSides=3  GraphicOpacity=1.0  PolygonOuterRadius=1  PolygonOuterRadiusUnits=m  ProductsOfInertia=[0 0 0]  ProductsOfInertiaUnits=kg*m^2  GraphicShininess=75  GraphicSpecularColor=[0.5 0.5 0.5 1.0]  GraphicVisPropType=SimpleVisualProperties
  Carrier Shaft Hole : sm_robotic_wrist_lib/Plate with Hole  L=4*Rhc  W=Wc  T=Tc  Rh=Rhc  rho=rho  clr=cclr  opc=1
      settings: SourceProductBaseCode=MS
  Gear : sm_robotic_wrist_lib/Bevel Gear  R=Rg  T=Tg  Ca=Ag  Rh=Rgh  rho=rho  clr=gclr
      settings: SourceProductBaseCode=MS
  Gear XForm : sm_lib/Frames and Transforms/Rigid Transform  TranslationMethod=StandardAxis  TranslationStandardOffset=Tg/2  TranslationLengthUnit=cm  TranslationStandardAxis=-Y  TranslationCartesianOffset=[0 0 0]  TranslationROffset=0  TranslationROffsetUnits=m  TranslationZOffset=0  TranslationZOffsetUnits=m  TranslationThetaOffset=0  TranslationThetaOffsetUnits=deg  RotationMethod=AlignedAxes  RotationAngleUnits=deg  RotationStandardAxis=+Z  RotationAngle=0  RotationArbitraryAxis=[0 0 1]  FollAlignAxisA=+Z  BaseAlignAxisA=-Y  FollAlignAxisB=+X  BaseAlignAxisB=+X  RotationSequenceAxes=FollowerAxes  RotationSequence=XYX  RotationSequenceAngles=[0 0 0]  RotationSequenceAnglesUnits=deg  RotationMatrix=[1 0 0; 0 1 0; 0 0 1]
  RB XForm 1 : sm_lib/Frames and Transforms/Rigid Transform  TranslationMethod=Cartesian  TranslationStandardOffset=0  TranslationLengthUnit=cm  TranslationStandardAxis=+Z  TranslationCartesianOffset=[rhx rhy 0]  TranslationROffset=0  TranslationROffsetUnits=m  TranslationZOffset=0  TranslationZOffsetUnits=m  TranslationThetaOffset=0  TranslationThetaOffsetUnits=deg  RotationMethod=StandardAxis  RotationAngleUnits=deg  RotationStandardAxis=+Z  RotationAngle=90-Ac  RotationArbitraryAxis=[0 0 1]  FollAlignAxisA=+X  BaseAlignAxisA=+Y  FollAlignAxisB=+Y  BaseAlignAxisB=+Z  RotationSequenceAxes=FollowerAxes  RotationSequence=XYX  RotationSequenceAngles=[0 0 0]  RotationSequenceAnglesUnits=deg  RotationMatrix=[1 0 0; 0 1 0; 0 0 1]
  RB XForm 2 : sm_lib/Frames and Transforms/Rigid Transform  TranslationMethod=StandardAxis  TranslationStandardOffset=Tc/2  TranslationLengthUnit=cm  TranslationStandardAxis=+X  TranslationCartesianOffset=[0 0 0]  TranslationROffset=0  TranslationROffsetUnits=m  TranslationZOffset=0  TranslationZOffsetUnits=m  TranslationThetaOffset=0  TranslationThetaOffsetUnits=deg  RotationMethod=AlignedAxes  RotationAngleUnits=deg  RotationStandardAxis=+Z  RotationAngle=0  RotationArbitraryAxis=[0 0 1]  FollAlignAxisA=+Z  BaseAlignAxisA=+X  FollAlignAxisB=+X  BaseAlignAxisB=-Y  RotationSequenceAxes=FollowerAxes  RotationSequence=XYX  RotationSequenceAngles=[0 0 0]  RotationSequenceAnglesUnits=deg  RotationMatrix=[1 0 0; 0 1 0; 0 0 1]
  TB XForm : sm_lib/Frames and Transforms/Rigid Transform  TranslationMethod=StandardAxis  TranslationStandardOffset=Hc-Tc/2  TranslationLengthUnit=cm  TranslationStandardAxis=+Y  TranslationCartesianOffset=[0 0 0]  TranslationROffset=0  TranslationROffsetUnits=m  TranslationZOffset=0  TranslationZOffsetUnits=m  TranslationThetaOffset=0  TranslationThetaOffsetUnits=deg  RotationMethod=AlignedAxes  RotationAngleUnits=deg  RotationStandardAxis=+Z  RotationAngle=0  RotationArbitraryAxis=[0 0 1]  FollAlignAxisA=+Z  BaseAlignAxisA=+Y  FollAlignAxisB=+X  BaseAlignAxisB=+X  RotationSequenceAxes=FollowerAxes  RotationSequence=XYX  RotationSequenceAngles=[0 0 0]  RotationSequenceAnglesUnits=deg  RotationMatrix=[1 0 0; 0 1 0; 0 0 1]
  Tool Shaft Hole : sm_robotic_wrist_lib/Plate with Hole  L=4*Rhc  W=Wc  T=Tc  Rh=Rhc  rho=rho  clr=cclr  opc=1
      settings: SourceProductBaseCode=MS
  G : PMIOPort  Side=Right
  HC : PMIOPort  Port=2  Side=Right
  HT : PMIOPort  Port=3  Side=Right
  connections:
  Carrier Shaft Hole/LConn1 -- TB XForm/RConn1 -- HC/RConn1
  TB XForm/LConn1 -- Carrier Right Top/RConn1 -- Gear XForm/LConn1 -- Carrier Left/RConn1 -- Carrier Right Bottom/RConn1 -- RB XForm 1/LConn1
  RB XForm 1/RConn1 -- RB XForm 2/LConn1
  Tool Shaft Hole/LConn1 -- HT/RConn1 -- RB XForm 2/RConn1
  G/RConn1 -- Gear/LConn1 -- Gear XForm/RConn1

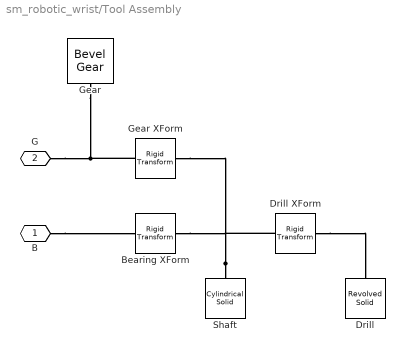
== system sm_robotic_wrist/Tool Assembly ==
  Bearing XForm : sm_lib/Frames and Transforms/Rigid Transform  TranslationMethod=StandardAxis  TranslationStandardOffset=L/2-Oh-Tg/2  TranslationLengthUnit=cm  TranslationStandardAxis=-Z  TranslationCartesianOffset=[0 0 0]  TranslationROffset=0  TranslationROffsetUnits=m  TranslationZOffset=0  TranslationZOffsetUnits=m  TranslationThetaOffset=0  TranslationThetaOffsetUnits=deg  RotationMethod=None  RotationAngleUnits=deg  RotationStandardAxis=+Z  RotationAngle=0  RotationArbitraryAxis=[0 0 1]  FollAlignAxisA=+Z  BaseAlignAxisA=-Z  FollAlignAxisB=+X  BaseAlignAxisB=+X  RotationSequenceAxes=FollowerAxes  RotationSequence=XYX  RotationSequenceAngles=[0 0 0]  RotationSequenceAnglesUnits=deg  RotationMatrix=[1 0 0; 0 1 0; 0 0 1]
  Drill : sm_lib/Body Elements/Revolved Solid  GraphicAmbientColor=[0.15 0.15 0.15 1.0]  BasedOnType=Density  CenterOfMass=[0 0 0]  CenterOfMassUnits=m  GraphicDiffuseColor=clr  ExportConvexHullGeometry=off  Density=rho  DensityUnits=kg/(m^3)  DoExposeReferenceFrame=on  GraphicEmissiveColor=[0.0 0.0 0.0 1.0]  ExportEntireGeometry=off  SerializedFrames=<Frames/>  MarkerShape=Sphere  MarkerSize=10  GraphicType=FromGeometry  InertiaType=CalculateFromGeometry  Mass=1  MassUnits=kg  MomentsOfInertia=[1 1 1]  MomentsOfInertiaUnits=kg*m^2  GraphicOpacity=1.0  ProductsOfInertia=[0 0 0]  ProductsOfInertiaUnits=kg*m^2  RevolutionCrossSection=drill_xsec  RevolutionCrossSectionUnits=cm  RevolutionAngle=240  RevolutionAngleUnits=deg  RevolutionExtent=Custom  GraphicShininess=75  GraphicSpecularColor=[0.5 0.5 0.5 1.0]  GraphicVisPropType=SimpleVisualProperties
  Drill XForm : sm_lib/Frames and Transforms/Rigid Transform  TranslationMethod=StandardAxis  TranslationStandardOffset=L/2  TranslationLengthUnit=cm  TranslationStandardAxis=+Z  TranslationCartesianOffset=[0 0 0]  TranslationROffset=0  TranslationROffsetUnits=m  TranslationZOffset=0  TranslationZOffsetUnits=m  TranslationThetaOffset=0  TranslationThetaOffsetUnits=deg  RotationMethod=None  RotationAngleUnits=deg  RotationStandardAxis=+Z  RotationAngle=0  RotationArbitraryAxis=[0 0 1]  FollAlignAxisA=+Z  BaseAlignAxisA=+Y  FollAlignAxisB=+X  BaseAlignAxisB=-X  RotationSequenceAxes=FollowerAxes  RotationSequence=XYX  RotationSequenceAngles=[0 0 0]  RotationSequenceAnglesUnits=deg  RotationMatrix=[1 0 0; 0 1 0; 0 0 1]
  Gear : sm_robotic_wrist_lib/Bevel Gear  R=Rg  T=Tg  Ca=Cag  Rh=R  rho=rho  clr=clr
      settings: SourceProductBaseCode=MS
  Gear XForm : sm_lib/Frames and Transforms/Rigid Transform  TranslationMethod=StandardAxis  TranslationStandardOffset=L/2-Tg/2  TranslationLengthUnit=cm  TranslationStandardAxis=-Z  TranslationCartesianOffset=[0 0 0]  TranslationROffset=0  TranslationROffsetUnits=m  TranslationZOffset=0  TranslationZOffsetUnits=m  TranslationThetaOffset=0  TranslationThetaOffsetUnits=deg  RotationMethod=AlignedAxes  RotationAngleUnits=deg  RotationStandardAxis=+Z  RotationAngle=0  RotationArbitraryAxis=[0 0 1]  FollAlignAxisA=+Z  BaseAlignAxisA=-Z  FollAlignAxisB=+X  BaseAlignAxisB=+X  RotationSequenceAxes=FollowerAxes  RotationSequence=XYX  RotationSequenceAngles=[0 0 0]  RotationSequenceAnglesUnits=deg  RotationMatrix=[1 0 0; 0 1 0; 0 0 1]
  Shaft : sm_lib/Body Elements/Cylindrical Solid  GraphicAmbientColor=[0.15 0.15 0.15 1.0]  BasedOnType=Density  CenterOfMass=[0 0 0]  CenterOfMassUnits=m  GraphicDiffuseColor=clr  CylinderLength=L  CylinderLengthUnits=cm  CylinderRadius=R  CylinderRadiusUnits=cm  Density=rho  DensityUnits=kg/(m^3)  DoExposeReferenceFrame=on  GraphicEmissiveColor=[0.0 0.0 0.0 1.0]  ExportEntireGeometry=off  SerializedFrames=<Frames/>  MarkerShape=Sphere  MarkerSize=10  GraphicType=FromGeometry  InertiaType=CalculateFromGeometry  Mass=1  MassUnits=kg  MomentsOfInertia=[1 1 1]  MomentsOfInertiaUnits=kg*m^2  GraphicOpacity=1.0  ProductsOfInertia=[0 0 0]  ProductsOfInertiaUnits=kg*m^2  GraphicShininess=75  GraphicSpecularColor=[0.5 0.5 0.5 1.0]  GraphicVisPropType=SimpleVisualProperties
  B : PMIOPort  Side=Left
  G : PMIOPort  Port=2  Side=Left
  connections:
  G/RConn1 -- Gear XForm/RConn1 -- Gear/LConn1
  Shaft/RConn1 -- Drill XForm/LConn1 -- Gear XForm/LConn1 -- Bearing XForm/LConn1
  Drill XForm/RConn1 -- Drill/RConn1
  B/RConn1 -- Bearing XForm/RConn1

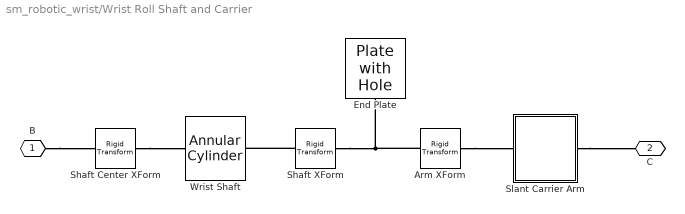
== system sm_robotic_wrist/Wrist Roll Shaft and Carrier ==
  Arm XForm : sm_lib/Frames and Transforms/Rigid Transform  TranslationMethod=StandardAxis  TranslationStandardOffset=wshaft.Lep/2  TranslationLengthUnit=cm  TranslationStandardAxis=+X  TranslationCartesianOffset=[0 0 0]  TranslationROffset=0  TranslationROffsetUnits=m  TranslationZOffset=0  TranslationZOffsetUnits=m  TranslationThetaOffset=0  TranslationThetaOffsetUnits=deg  RotationMethod=AlignedAxes  RotationAngleUnits=deg  RotationStandardAxis=+Z  RotationAngle=0  RotationArbitraryAxis=[0 0 1]  FollAlignAxisA=+Z  BaseAlignAxisA=-X  FollAlignAxisB=+Y  BaseAlignAxisB=+Y  RotationSequenceAxes=FollowerAxes  RotationSequence=XYX  RotationSequenceAngles=[0 0 0]  RotationSequenceAnglesUnits=deg  RotationMatrix=[1 0 0; 0 1 0; 0 0 1]
  End Plate : sm_robotic_wrist_lib/Plate with Hole  L=wshaft.Lep  W=wshaft.Lep  T=wshaft.Tep  Rh=wshaft.Rsi  rho=density.aluminum  clr=color.orange  opc=1
      settings: SourceProductBaseCode=MS
  Shaft Center XForm : sm_lib/Frames and Transforms/Rigid Transform  TranslationMethod=StandardAxis  TranslationStandardOffset=wshaft.Ls/2  TranslationLengthUnit=cm  TranslationStandardAxis=+Z  TranslationCartesianOffset=[0 0 0]  TranslationROffset=0  TranslationROffsetUnits=m  TranslationZOffset=0  TranslationZOffsetUnits=m  TranslationThetaOffset=0  TranslationThetaOffsetUnits=deg  RotationMethod=None  RotationAngleUnits=deg  RotationStandardAxis=+Z  RotationAngle=0  RotationArbitraryAxis=[0 0 1]  FollAlignAxisA=+X  BaseAlignAxisA=+Y  FollAlignAxisB=+Y  BaseAlignAxisB=+Z  RotationSequenceAxes=FollowerAxes  RotationSequence=XYX  RotationSequenceAngles=[0 0 0]  RotationSequenceAnglesUnits=deg  RotationMatrix=[1 0 0; 0 1 0; 0 0 1]
  Shaft XForm : sm_lib/Frames and Transforms/Rigid Transform  TranslationMethod=StandardAxis  TranslationStandardOffset=wshaft.Tep/2  TranslationLengthUnit=cm  TranslationStandardAxis=-Z  TranslationCartesianOffset=[0 0 0]  TranslationROffset=0  TranslationROffsetUnits=m  TranslationZOffset=0  TranslationZOffsetUnits=m  TranslationThetaOffset=0  TranslationThetaOffsetUnits=deg  RotationMethod=None  RotationAngleUnits=deg  RotationStandardAxis=+Z  RotationAngle=0  RotationArbitraryAxis=[0 0 1]  FollAlignAxisA=+Z  BaseAlignAxisA=+X  FollAlignAxisB=+Y  BaseAlignAxisB=+Y  RotationSequenceAxes=FollowerAxes  RotationSequence=XYX  RotationSequenceAngles=[0 0 0]  RotationSequenceAnglesUnits=deg  RotationMatrix=[1 0 0; 0 1 0; 0 0 1]
  Slant Carrier Arm : Subsystem  mask(Slant Arm with Hole){L=wshaft.Lsa, W=wshaft.Lep, T=wshaft.Tep, Rh=wshaft.Rhsa, Oh=wshaft.Oh, Sa=Ca, rho=density.aluminum, clr=color.orange, opc=1}
      mask prompts: L "Length (cm):"; W "Width (cm):"; T "Thickness (cm):"; Rh "Hole radius (cm):"; Oh "Hole offset (cm):"; Sa "Slant edge angle (deg):"; rho "Density (kg/m^3)"; clr "Color"; opc "Opacity"
      mask help:
      | This block models a slant arm with a hole at the bottom.
      |
      | The port T corresponds to the frame at the center of the top face of the arm.
      |
      | The port H corresponds to the center of the hole.
      mask init:
      | plate_xsec = [Oh 0; Oh W/2; -(L-Oh) W/2; 
      |              -(L-Oh) -W/2; Oh -W/2; Oh 0];
      | th = linspace(360,0,360)'*pi/180;          
      | plate_xsec = [plate_xsec; Rh*cos(th) Rh*sin(th)];
      mask DialogControl Container4 Prompt: Dimensions
      mask DialogControl Container4_copy Prompt: Material Properties
      mask Display:
      | image(fullfile(matlabroot,'toolbox','physmod','sm','smdemos','robotic_wrist','images','sm_rwrist_slantarm.png'))
      | port_label('LConn',1,'T')
      | port_label('RConn',1,'H')
  Wrist Shaft : sm_robotic_wrist_lib/Annular Cylinder  Ro=wshaft.Rso  Ri=wshaft.Rsi  L=wshaft.Ls  rho=density.aluminum  clr=color.orange  opc=1
      settings: SourceProductBaseCode=MS
  B : PMIOPort  Side=Left
  C : PMIOPort  Port=2  Side=Right
  connections:
  Slant Carrier Arm/RConn1 -- C/RConn1
  Shaft Center XForm/LConn1 -- Wrist Shaft/LConn1
  B/RConn1 -- Shaft Center XForm/RConn1
  Shaft XForm/RConn1 -- Wrist Shaft/RConn1
  Shaft XForm/LConn1 -- Arm XForm/LConn1 -- End Plate/LConn1
  Arm XForm/RConn1 -- Slant Carrier Arm/LConn1

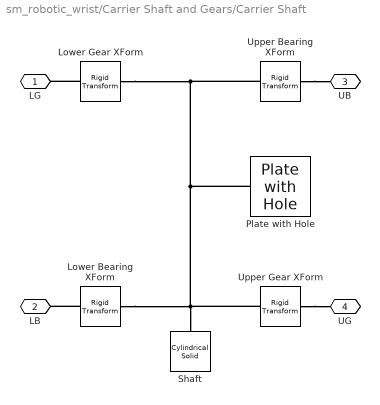
== system sm_robotic_wrist/Carrier Shaft and Gears/Carrier Shaft ==
  Lower Bearing XForm : sm_lib/Frames and Transforms/Rigid Transform  TranslationMethod=StandardAxis  TranslationStandardOffset=Ohl  TranslationLengthUnit=cm  TranslationStandardAxis=-Z  TranslationCartesianOffset=[0 0 0]  TranslationROffset=0  TranslationROffsetUnits=m  TranslationZOffset=0  TranslationZOffsetUnits=m  TranslationThetaOffset=0  TranslationThetaOffsetUnits=deg  RotationMethod=None  RotationAngleUnits=deg  RotationStandardAxis=+Z  RotationAngle=0  RotationArbitraryAxis=[0 0 1]  FollAlignAxisA=+X  BaseAlignAxisA=+Y  FollAlignAxisB=+Y  BaseAlignAxisB=+Z  RotationSequenceAxes=FollowerAxes  RotationSequence=XYX  RotationSequenceAngles=[0 0 0]  RotationSequenceAnglesUnits=deg  RotationMatrix=[1 0 0; 0 1 0; 0 0 1]
  Lower Gear XForm : sm_lib/Frames and Transforms/Rigid Transform  TranslationMethod=StandardAxis  TranslationStandardOffset=Og  TranslationLengthUnit=cm  TranslationStandardAxis=-Z  TranslationCartesianOffset=[0 0 0]  TranslationROffset=0  TranslationROffsetUnits=m  TranslationZOffset=0  TranslationZOffsetUnits=m  TranslationThetaOffset=0  TranslationThetaOffsetUnits=deg  RotationMethod=None  RotationAngleUnits=deg  RotationStandardAxis=+Z  RotationAngle=0  RotationArbitraryAxis=[0 0 1]  FollAlignAxisA=+X  BaseAlignAxisA=+Y  FollAlignAxisB=+Y  BaseAlignAxisB=+Z  RotationSequenceAxes=FollowerAxes  RotationSequence=XYX  RotationSequenceAngles=[0 0 0]  RotationSequenceAnglesUnits=deg  RotationMatrix=[1 0 0; 0 1 0; 0 0 1]
  Plate with Hole : sm_robotic_wrist_lib/Plate with Hole  L=2.5*R  W=2.5*R  T=L/4  Rh=R  rho=rho  clr=0.5*clr  opc=1
      settings: SourceProductBaseCode=MS
  Shaft : sm_lib/Body Elements/Cylindrical Solid  GraphicAmbientColor=[0.15 0.15 0.15 1.0]  BasedOnType=Density  CenterOfMass=[0 0 0]  CenterOfMassUnits=m  GraphicDiffuseColor=clr  CylinderLength=L  CylinderLengthUnits=cm  CylinderRadius=R  CylinderRadiusUnits=cm  Density=rho  DensityUnits=kg/(m^3)  DoExposeReferenceFrame=on  GraphicEmissiveColor=[0.0 0.0 0.0 1.0]  ExportEntireGeometry=off  SerializedFrames=<Frames/>  MarkerShape=Sphere  MarkerSize=10  GraphicType=FromGeometry  InertiaType=CalculateFromGeometry  Mass=1  MassUnits=kg  MomentsOfInertia=[1 1 1]  MomentsOfInertiaUnits=kg*m^2  GraphicOpacity=1.0  ProductsOfInertia=[0 0 0]  ProductsOfInertiaUnits=kg*m^2  GraphicShininess=75  GraphicSpecularColor=[0.5 0.5 0.5 1.0]  GraphicVisPropType=SimpleVisualProperties
  Upper Bearing XForm : sm_lib/Frames and Transforms/Rigid Transform  TranslationMethod=StandardAxis  TranslationStandardOffset=Ohu  TranslationLengthUnit=cm  TranslationStandardAxis=+Z  TranslationCartesianOffset=[0 0 0]  TranslationROffset=0  TranslationROffsetUnits=m  TranslationZOffset=0  TranslationZOffsetUnits=m  TranslationThetaOffset=0  TranslationThetaOffsetUnits=deg  RotationMethod=None  RotationAngleUnits=deg  RotationStandardAxis=+Z  RotationAngle=0  RotationArbitraryAxis=[0 0 1]  FollAlignAxisA=+X  BaseAlignAxisA=+Y  FollAlignAxisB=+Y  BaseAlignAxisB=+Z  RotationSequenceAxes=FollowerAxes  RotationSequence=XYX  RotationSequenceAngles=[0 0 0]  RotationSequenceAnglesUnits=deg  RotationMatrix=[1 0 0; 0 1 0; 0 0 1]
  Upper Gear XForm : sm_lib/Frames and Transforms/Rigid Transform  TranslationMethod=StandardAxis  TranslationStandardOffset=Og  TranslationLengthUnit=cm  TranslationStandardAxis=+Z  TranslationCartesianOffset=[0 0 0]  TranslationROffset=0  TranslationROffsetUnits=m  TranslationZOffset=0  TranslationZOffsetUnits=m  TranslationThetaOffset=0  TranslationThetaOffsetUnits=deg  RotationMethod=AlignedAxes  RotationAngleUnits=deg  RotationStandardAxis=+Z  RotationAngle=0  RotationArbitraryAxis=[0 0 1]  FollAlignAxisA=+Z  BaseAlignAxisA=-Z  FollAlignAxisB=+X  BaseAlignAxisB=+X  RotationSequenceAxes=FollowerAxes  RotationSequence=XYX  RotationSequenceAngles=[0 0 0]  RotationSequenceAnglesUnits=deg  RotationMatrix=[1 0 0; 0 1 0; 0 0 1]
  LG : PMIOPort  Side=Left
  LB : PMIOPort  Port=2  Side=Left
  UB : PMIOPort  Port=3  Side=Right
  UG : PMIOPort  Port=4  Side=Right
  connections:
  Lower Bearing XForm/RConn1 -- LB/RConn1
  Upper Bearing XForm/RConn1 -- UB/RConn1
  Lower Gear XForm/RConn1 -- LG/RConn1
  Lower Bearing XForm/LConn1 -- Upper Bearing XForm/LConn1 -- Lower Gear XForm/LConn1 -- Plate with Hole/LConn1 -- Upper Gear XForm/LConn1 -- Shaft/RConn1
  Upper Gear XForm/RConn1 -- UG/RConn1
